simulink model "All_Controller_Compare_Angle_Disturbance"  (R2022a)
settings: Solver=VariableStepAuto  StartTime=0.0  StopTime=130  RelTol=1e-3
undefined symbols (not defined in the file): A, att_opt, B, C, ki_u4_, Klqr, L, pitch_opt, roll_opt, x_opt, y_opt, yaw_opt
libraries: slpidlib x6, simulink x2
settings Model: Creator=creec  LastModifiedBy=creec

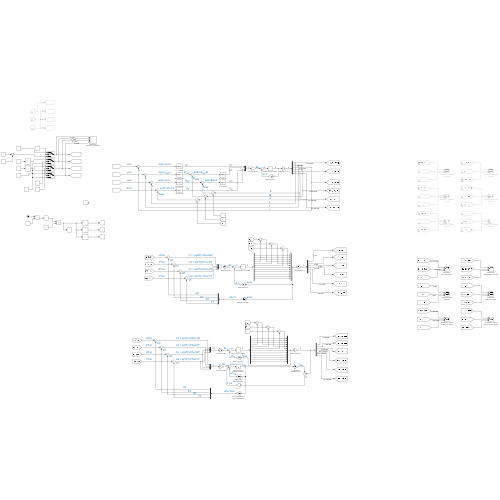
[thumbnail: Simulink's stored preview of the top-level diagram]
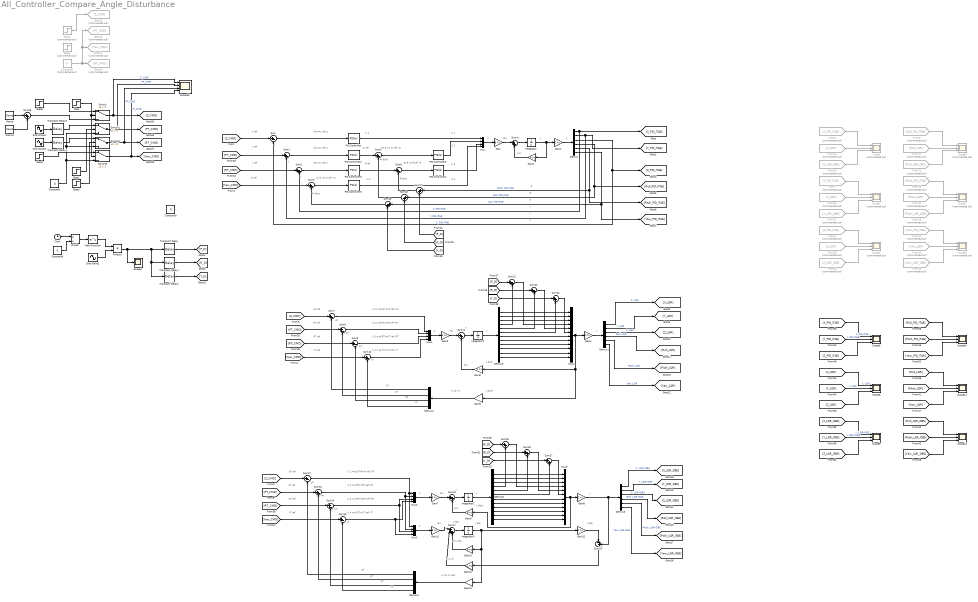
== system All_Controller_Compare_Angle_Disturbance ==
  note: z
  note: x ref
  note: U 1
  note: U 4
  note: x
  note: Ψ distr
  note: x'
  note: θ
  note: Ψ ref
  note: e(y)=y ref -y
  note: e(x)=x ref -x
  note: U 1
  note: e( θ )= θ ref - θ
  note: Φ ref
  note: x
  note: x
  note: Ψ
  note: A*x
  note: e(z)=z ref -z
  note: y
  note: U 2
  note: U
  note: z
  note: θ distr
  note: Bu
  note: U 4
  note: Φ distr
  note: Φ
  note: y ref
  note: y
  note: y
  note: z ref
  note: e( Ψ )= Ψ ref - Ψ
  note: U 3
  note: θ ref
  note: e( Φ )= Φ ref - Φ
  note: PT
  note: y
  note: U 3 = e(RT)=RT ref -RT
  note: U 4 = e(YT)=YT ref -YT
  note: U 2 = e(PT)=PT ref -PT
  note: x distr
  note: RT
  note: PT
  note: - K lqr *x
  note: UF
  note: Bu
  note: UF ref
  note: U 1 = e(UF)=UF ref -UF
  note: RT ref
  note: x
  note: UF
  note: A*x
  note: YT ref
  note: PT ref
  note: U
  note: x'
  note: YT
  note: RT
  note: YT
  note: x obs
  note: L*y e
  note: RT ref
  note: YT ref
  note: x
  note: U
  note: YT
  note: U 1 = e(UF)=UF ref -UF
  note: x'
  note: A*x
  note: YT
  note: A*x obs
  note: PT ref
  note: UF
  note: U
  note: UF
  note: UF ref
  note: Bu
  note: RT
  note: U 2 = e(PT)=PT ref -PT
  note: RT
  note: U 4 = e(YT)=YT ref -YT
  note: x obs '
  note: PT
  note: U 3 = e(RT)=RT ref -RT
  note: PT
  note: y e
  note: - K lqr *x obs
  note: y
  note: y obs
  note: Bu
  note: x distr
  note: x distr
  Clock : Clock
  Constant1 : Constant  Value=0
  Constant6 : Constant  Commented=on  Value=0
  Constant8 : Constant  Value=-1  SampleTime=-1
  Constant9 : Constant  Value=0
  Demux : Demux  Outputs=6
  Demux1 : Demux  Outputs=6
  Demux2 : Demux
  Demux3 : Demux  Outputs=6
  Demux4 : Demux
  Demux5 : Demux  Outputs=12
  Demux6 : Demux  Outputs=12
  Divide : Product  Inputs=*/
  From10 : From  Commented=on  GotoTag=Pitch_PID_ITAE
  From11 : From  Commented=on  GotoTag=Yaw_PID_ITAE
  From12 : From  Commented=on  GotoTag=Pitch_LQR
  From13 : From  Commented=on  GotoTag=Yaw_LQR
  From14 : From  Commented=on  GotoTag=X_LQR
  From15 : From  Commented=on  GotoTag=Y_LQR
  From16 : From  Commented=on  GotoTag=Z_LQR
  From17 : From  Commented=on  GotoTag=Roll_LQR
  From18 : From  Commented=on  GotoTag=Pitch_LQR_OBS
  From19 : From  Commented=on  GotoTag=Yaw_LQR_OBS
  From20 : From  Commented=on  GotoTag=X_LQR_OBS
  From21 : From  Commented=on  GotoTag=Y_LQR_OBS
  From22 : From  Commented=on  GotoTag=Z_LQR_OBS
  From23 : From  Commented=on  GotoTag=Roll_LQR_OBS
  From6 : From  Commented=on  GotoTag=X_PID_ITAE
  From7 : From  Commented=on  GotoTag=Y_PID_ITAE
  From8 : From  Commented=on  GotoTag=Z_PID_ITAE
  From9 : From  Commented=on  GotoTag=Roll_PID_ITAE
  Gain{,3,7,11} (4 alike) : Gain  Gain=B  Multiplication=Matrix(K*u)
      settings: AttributesFormatString=State-Space B*u
  Gain{1,4,8,12} (4 alike) : Gain  Gain=C  Multiplication=Matrix(K*u)
      Gain1 settings: AttributesFormatString=State-Space C*x
      Gain12 settings: AttributesFormatString=|
      | Augmented
      | State-Space C*x
      Gain4 settings: AttributesFormatString=State-Space C*x
      Gain8 settings: AttributesFormatString=State-Space C*x
  Gain10 : Gain  Gain=Klqr  Multiplication=Matrix(K*u)
      settings: AttributesFormatString=|
      | LQR Feedback Gain,
      | Augmented States
  Gain{2,5,9,13} (4 alike) : Gain  Gain=A  Multiplication=Matrix(K*u)
      Gain13 settings: AttributesFormatString=|
      | Augmented
      | State-Space A*x
      Gain2 settings: AttributesFormatString=State-Space A*x
      Gain5 settings: AttributesFormatString=State-Space A*x
      Gain9 settings: AttributesFormatString=State-Space A*x
  Gain14 : Gain  Gain=L  Multiplication=Matrix(K*u)
      settings: AttributesFormatString=L*y_e
  Gain6 : Gain  Gain=Klqr  Multiplication=Matrix(K*u)
      settings: AttributesFormatString=LQR Feeback Gain
  Goto21 : Goto  Commented=on  GotoTag=Yaw_CMD
  Goto23 : Goto  Commented=on  GotoTag=PT_CMD
  Goto24 : Goto  Commented=on  GotoTag=RT_CMD
  Goto25 : Goto  Commented=on  GotoTag=Z_CMD
  Integrator{,1..3} (4 alike) : Integrator
      Integrator settings: AttributesFormatString=Extract Current States
      Integrator1 settings: AttributesFormatString=Extract Current States
      Integrator2 settings: AttributesFormatString=Extract Current States
      Integrator3 settings: AttributesFormatString=|
      | Extract Current
      | Augmented States
  Math Function : Math
  Mux{,1..3} (4 alike) : Mux
  Mux4 : Mux  Inputs=12
  Mux5 : Mux  Inputs=12
  PID Controller : slpidlib/PID Controller  Controller=PID  Form=Parallel  TimeDomain=Continuous-time  UseExternalTs=off  SampleTime=-1  IntegratorMethod=Forward Euler  FilterMethod=Forward Euler  ControllerParametersSource=internal  P=att_opt(1)  I=att_opt(2)  UseKiTs=off  D=att_opt(3)  N=100  UseFilter=on  TunerSelectOption=Transfer Function Based (PID Tuner App)  InitialConditionSource=internal  InitialConditionForIntegrator=0  InitialConditionForFilter=0  DifferentiatorICPrevScaledInput=0  ExternalReset=none  TrackingMode=off  Kt=1  LimitOutput=off  SatLimitsSource=internal  UpperSaturationLimit=inf  LowerSaturationLimit=-inf  LinearizeAsGain=on  AntiWindupMode=none  Kb=1  POutMin=[]  POutMax=[]  IOutMin=[]  IOutMax=[]  DOutMin=[]  DOutMax=[]  NOutMin=[]  NOutMax=[]  SumOutMin=[]  SumOutMax=[]  SaturationOutMin=[]  SaturationOutMax=[]  PParamMin=[]  PParamMax=[]  IParamMin=[]  IParamMax=[]  DParamMin=[]  DParamMax=[]  NParamMin=[]  NParamMax=[]  KbParamMin=[]  KbParamMax=[]  KtParamMin=[]  KtParamMax=[]  KbOutMin=[]  KbOutMax=[]  KtOutMin=[]  KtOutMax=[]  IntegratorOutMin=[]  IntegratorOutMax=[]  FilterOutMin=[]  FilterOutMax=[]  SumI1OutMin=[]  SumI1OutMax=[]  SumI2OutMin=[]  SumI2OutMax=[]  SumI3OutMin=[]  SumI3OutMax=[]  SumI4OutMin=[]  SumI4OutMax=[]  SumDOutMin=[]  SumDOutMax=[]  DifferentiatorOutMin=[]  DifferentiatorOutMax=[]  FilterDiffOutCoefMin=[]  FilterDiffOutCoefMax=[]  ReciprocalOutMin=[]  ReciprocalOutMax=[]  SumDenOutMin=[]  SumDenOutMax=[]  SumNumOutMin=[]  SumNumOutMax=[]  DivideOutMin=[]  DivideOutMax=[]  UdiffTsProdOutMin=[]  UdiffTsProdOutMax=[]  NTsProdOutMin=[]  NTsProdOutMax=[]  UintegralTsProdOutMin=[]  UintegralTsProdOutMax=[]  UngainTsProdOutMin=[]  UngainTsProdOutMax=[]  IntegratorContinuousStateAttributes=''  IntegratorStateMustResolveToSignalObject=off  IntegratorRTWStateStorageClass=Auto  FilterContinuousStateAttributes=''  FilterStateMustResolveToSignalObject=off  FilterRTWStateStorageClass=Auto  ParallelPVariant=InternalParameters  IdealPVariant=Disabled  IVariant=InternalParameters  DVariant=InternalParameters  IntegratorVariant=Continuous  SatVariant=Disabled  AWVariant=Passthrough  PCopyVariant=Disabled  TRVariant=Disabled  FdbkBlocksVariant=Forward  IdealPFdbkVariant=Disabled  SatFdbkVariant=Disabled  DerivativeFilterVariant=ContFilter  NVariant=InternalParameters  NCopyVariant=Disabled  FilterICVariant=InternalICsFilter  IntegratorICVariant=InternalICs  ExternalResetVariant=Disabled  TRSumVariant=Passthrough  SumFdbkVariant=Disabled  SumVariant=Sum_PID  TsampFilterVariant=InternalTs  TsampNgainVariant=Passthrough  TsampIntegralVariant=Passthrough  ExternalSaturationOutDataTypeStr=Inherit: Same as second input  aMode=0
      settings: AttributesFormatString=U1 Controller
  PID Controller1 : slpidlib/PID Controller  Controller=PD  Form=Parallel  TimeDomain=Continuous-time  UseExternalTs=off  SampleTime=-1  IntegratorMethod=Forward Euler  FilterMethod=Forward Euler  ControllerParametersSource=internal  P=y_opt(1)  I=0  UseKiTs=off  D=y_opt(2)  N=100  UseFilter=on  TunerSelectOption=Transfer Function Based (PID Tuner App)  InitialConditionSource=internal  InitialConditionForIntegrator=0  InitialConditionForFilter=0  DifferentiatorICPrevScaledInput=0  ExternalReset=none  TrackingMode=off  Kt=1  LimitOutput=off  SatLimitsSource=internal  UpperSaturationLimit=inf  LowerSaturationLimit=-inf  LinearizeAsGain=on  AntiWindupMode=none  Kb=1  POutMin=[]  POutMax=[]  IOutMin=[]  IOutMax=[]  DOutMin=[]  DOutMax=[]  NOutMin=[]  NOutMax=[]  SumOutMin=[]  SumOutMax=[]  SaturationOutMin=[]  SaturationOutMax=[]  PParamMin=[]  PParamMax=[]  IParamMin=[]  IParamMax=[]  DParamMin=[]  DParamMax=[]  NParamMin=[]  NParamMax=[]  KbParamMin=[]  KbParamMax=[]  KtParamMin=[]  KtParamMax=[]  KbOutMin=[]  KbOutMax=[]  KtOutMin=[]  KtOutMax=[]  IntegratorOutMin=[]  IntegratorOutMax=[]  FilterOutMin=[]  FilterOutMax=[]  SumI1OutMin=[]  SumI1OutMax=[]  SumI2OutMin=[]  SumI2OutMax=[]  SumI3OutMin=[]  SumI3OutMax=[]  SumI4OutMin=[]  SumI4OutMax=[]  SumDOutMin=[]  SumDOutMax=[]  DifferentiatorOutMin=[]  DifferentiatorOutMax=[]  FilterDiffOutCoefMin=[]  FilterDiffOutCoefMax=[]  ReciprocalOutMin=[]  ReciprocalOutMax=[]  SumDenOutMin=[]  SumDenOutMax=[]  SumNumOutMin=[]  SumNumOutMax=[]  DivideOutMin=[]  DivideOutMax=[]  UdiffTsProdOutMin=[]  UdiffTsProdOutMax=[]  NTsProdOutMin=[]  NTsProdOutMax=[]  UintegralTsProdOutMin=[]  UintegralTsProdOutMax=[]  UngainTsProdOutMin=[]  UngainTsProdOutMax=[]  IntegratorContinuousStateAttributes=''  IntegratorStateMustResolveToSignalObject=off  IntegratorRTWStateStorageClass=Auto  FilterContinuousStateAttributes=''  FilterStateMustResolveToSignalObject=off  FilterRTWStateStorageClass=Auto  ParallelPVariant=InternalParameters  IdealPVariant=Disabled  IVariant=Disabled  DVariant=InternalParameters  IntegratorVariant=Disabled  SatVariant=Disabled  AWVariant=Disabled  PCopyVariant=Disabled  TRVariant=Disabled  FdbkBlocksVariant=Forward  IdealPFdbkVariant=Disabled  SatFdbkVariant=Disabled  DerivativeFilterVariant=ContFilter  NVariant=InternalParameters  NCopyVariant=Disabled  FilterICVariant=InternalICsFilter  IntegratorICVariant=Disabled  ExternalResetVariant=Disabled  TRSumVariant=Passthrough  SumFdbkVariant=Disabled  SumVariant=Sum_PD  TsampFilterVariant=InternalTs  TsampNgainVariant=Passthrough  TsampIntegralVariant=Disabled_SignalSpec  ExternalSaturationOutDataTypeStr=Inherit: Same as second input  aMode=0
      settings: AttributesFormatString=Φref Generation
  PID Controller2 : slpidlib/PID Controller  Controller=PID  Form=Parallel  TimeDomain=Continuous-time  UseExternalTs=off  SampleTime=-1  IntegratorMethod=Forward Euler  FilterMethod=Forward Euler  ControllerParametersSource=internal  P=pitch_opt(1)  I=pitch_opt(2)  UseKiTs=off  D=pitch_opt(3)  N=100  UseFilter=on  TunerSelectOption=Transfer Function Based (PID Tuner App)  InitialConditionSource=internal  InitialConditionForIntegrator=0  InitialConditionForFilter=0  DifferentiatorICPrevScaledInput=0  ExternalReset=none  TrackingMode=off  Kt=1  LimitOutput=off  SatLimitsSource=internal  UpperSaturationLimit=inf  LowerSaturationLimit=-inf  LinearizeAsGain=on  AntiWindupMode=none  Kb=1  POutMin=[]  POutMax=[]  IOutMin=[]  IOutMax=[]  DOutMin=[]  DOutMax=[]  NOutMin=[]  NOutMax=[]  SumOutMin=[]  SumOutMax=[]  SaturationOutMin=[]  SaturationOutMax=[]  PParamMin=[]  PParamMax=[]  IParamMin=[]  IParamMax=[]  DParamMin=[]  DParamMax=[]  NParamMin=[]  NParamMax=[]  KbParamMin=[]  KbParamMax=[]  KtParamMin=[]  KtParamMax=[]  KbOutMin=[]  KbOutMax=[]  KtOutMin=[]  KtOutMax=[]  IntegratorOutMin=[]  IntegratorOutMax=[]  FilterOutMin=[]  FilterOutMax=[]  SumI1OutMin=[]  SumI1OutMax=[]  SumI2OutMin=[]  SumI2OutMax=[]  SumI3OutMin=[]  SumI3OutMax=[]  SumI4OutMin=[]  SumI4OutMax=[]  SumDOutMin=[]  SumDOutMax=[]  DifferentiatorOutMin=[]  DifferentiatorOutMax=[]  FilterDiffOutCoefMin=[]  FilterDiffOutCoefMax=[]  ReciprocalOutMin=[]  ReciprocalOutMax=[]  SumDenOutMin=[]  SumDenOutMax=[]  SumNumOutMin=[]  SumNumOutMax=[]  DivideOutMin=[]  DivideOutMax=[]  UdiffTsProdOutMin=[]  UdiffTsProdOutMax=[]  NTsProdOutMin=[]  NTsProdOutMax=[]  UintegralTsProdOutMin=[]  UintegralTsProdOutMax=[]  UngainTsProdOutMin=[]  UngainTsProdOutMax=[]  IntegratorContinuousStateAttributes=''  IntegratorStateMustResolveToSignalObject=off  IntegratorRTWStateStorageClass=Auto  FilterContinuousStateAttributes=''  FilterStateMustResolveToSignalObject=off  FilterRTWStateStorageClass=Auto  ParallelPVariant=InternalParameters  IdealPVariant=Disabled  IVariant=InternalParameters  DVariant=InternalParameters  IntegratorVariant=Continuous  SatVariant=Disabled  AWVariant=Passthrough  PCopyVariant=Disabled  TRVariant=Disabled  FdbkBlocksVariant=Forward  IdealPFdbkVariant=Disabled  SatFdbkVariant=Disabled  DerivativeFilterVariant=ContFilter  NVariant=InternalParameters  NCopyVariant=Disabled  FilterICVariant=InternalICsFilter  IntegratorICVariant=InternalICs  ExternalResetVariant=Disabled  TRSumVariant=Passthrough  SumFdbkVariant=Disabled  SumVariant=Sum_PID  TsampFilterVariant=InternalTs  TsampNgainVariant=Passthrough  TsampIntegralVariant=Passthrough  ExternalSaturationOutDataTypeStr=Inherit: Same as second input  aMode=0
      settings: AttributesFormatString=U2 Controller
  PID Controller3 : slpidlib/PID Controller  Controller=PD  Form=Parallel  TimeDomain=Continuous-time  UseExternalTs=off  SampleTime=-1  IntegratorMethod=Forward Euler  FilterMethod=Forward Euler  ControllerParametersSource=internal  P=x_opt(1)  I=-0.0096  UseKiTs=off  D=x_opt(2)  N=100  UseFilter=on  TunerSelectOption=Transfer Function Based (PID Tuner App)  InitialConditionSource=internal  InitialConditionForIntegrator=0  InitialConditionForFilter=0  DifferentiatorICPrevScaledInput=0  ExternalReset=none  TrackingMode=off  Kt=1  LimitOutput=off  SatLimitsSource=internal  UpperSaturationLimit=inf  LowerSaturationLimit=-inf  LinearizeAsGain=on  AntiWindupMode=none  Kb=1  POutMin=[]  POutMax=[]  IOutMin=[]  IOutMax=[]  DOutMin=[]  DOutMax=[]  NOutMin=[]  NOutMax=[]  SumOutMin=[]  SumOutMax=[]  SaturationOutMin=[]  SaturationOutMax=[]  PParamMin=[]  PParamMax=[]  IParamMin=[]  IParamMax=[]  DParamMin=[]  DParamMax=[]  NParamMin=[]  NParamMax=[]  KbParamMin=[]  KbParamMax=[]  KtParamMin=[]  KtParamMax=[]  KbOutMin=[]  KbOutMax=[]  KtOutMin=[]  KtOutMax=[]  IntegratorOutMin=[]  IntegratorOutMax=[]  FilterOutMin=[]  FilterOutMax=[]  SumI1OutMin=[]  SumI1OutMax=[]  SumI2OutMin=[]  SumI2OutMax=[]  SumI3OutMin=[]  SumI3OutMax=[]  SumI4OutMin=[]  SumI4OutMax=[]  SumDOutMin=[]  SumDOutMax=[]  DifferentiatorOutMin=[]  DifferentiatorOutMax=[]  FilterDiffOutCoefMin=[]  FilterDiffOutCoefMax=[]  ReciprocalOutMin=[]  ReciprocalOutMax=[]  SumDenOutMin=[]  SumDenOutMax=[]  SumNumOutMin=[]  SumNumOutMax=[]  DivideOutMin=[]  DivideOutMax=[]  UdiffTsProdOutMin=[]  UdiffTsProdOutMax=[]  NTsProdOutMin=[]  NTsProdOutMax=[]  UintegralTsProdOutMin=[]  UintegralTsProdOutMax=[]  UngainTsProdOutMin=[]  UngainTsProdOutMax=[]  IntegratorContinuousStateAttributes=''  IntegratorStateMustResolveToSignalObject=off  IntegratorRTWStateStorageClass=Auto  FilterContinuousStateAttributes=''  FilterStateMustResolveToSignalObject=off  FilterRTWStateStorageClass=Auto  ParallelPVariant=InternalParameters  IdealPVariant=Disabled  IVariant=Disabled  DVariant=InternalParameters  IntegratorVariant=Disabled  SatVariant=Disabled  AWVariant=Disabled  PCopyVariant=Disabled  TRVariant=Disabled  FdbkBlocksVariant=Forward  IdealPFdbkVariant=Disabled  SatFdbkVariant=Disabled  DerivativeFilterVariant=ContFilter  NVariant=InternalParameters  NCopyVariant=Disabled  FilterICVariant=InternalICsFilter  IntegratorICVariant=Disabled  ExternalResetVariant=Disabled  TRSumVariant=Passthrough  SumFdbkVariant=Disabled  SumVariant=Sum_PD  TsampFilterVariant=InternalTs  TsampNgainVariant=Passthrough  TsampIntegralVariant=Disabled_SignalSpec  ExternalSaturationOutDataTypeStr=Inherit: Same as second input  aMode=0
      settings: AttributesFormatString=θref Generation
  PID Controller4 : slpidlib/PID Controller  Controller=PID  Form=Parallel  TimeDomain=Continuous-time  UseExternalTs=off  SampleTime=-1  IntegratorMethod=Forward Euler  FilterMethod=Forward Euler  ControllerParametersSource=internal  P=roll_opt(1)  I=roll_opt(2)  UseKiTs=off  D=roll_opt(3)  N=100  UseFilter=on  TunerSelectOption=Transfer Function Based (PID Tuner App)  InitialConditionSource=internal  InitialConditionForIntegrator=0  InitialConditionForFilter=0  DifferentiatorICPrevScaledInput=0  ExternalReset=none  TrackingMode=off  Kt=1  LimitOutput=off  SatLimitsSource=internal  UpperSaturationLimit=inf  LowerSaturationLimit=-inf  LinearizeAsGain=on  AntiWindupMode=none  Kb=1  POutMin=[]  POutMax=[]  IOutMin=[]  IOutMax=[]  DOutMin=[]  DOutMax=[]  NOutMin=[]  NOutMax=[]  SumOutMin=[]  SumOutMax=[]  SaturationOutMin=[]  SaturationOutMax=[]  PParamMin=[]  PParamMax=[]  IParamMin=[]  IParamMax=[]  DParamMin=[]  DParamMax=[]  NParamMin=[]  NParamMax=[]  KbParamMin=[]  KbParamMax=[]  KtParamMin=[]  KtParamMax=[]  KbOutMin=[]  KbOutMax=[]  KtOutMin=[]  KtOutMax=[]  IntegratorOutMin=[]  IntegratorOutMax=[]  FilterOutMin=[]  FilterOutMax=[]  SumI1OutMin=[]  SumI1OutMax=[]  SumI2OutMin=[]  SumI2OutMax=[]  SumI3OutMin=[]  SumI3OutMax=[]  SumI4OutMin=[]  SumI4OutMax=[]  SumDOutMin=[]  SumDOutMax=[]  DifferentiatorOutMin=[]  DifferentiatorOutMax=[]  FilterDiffOutCoefMin=[]  FilterDiffOutCoefMax=[]  ReciprocalOutMin=[]  ReciprocalOutMax=[]  SumDenOutMin=[]  SumDenOutMax=[]  SumNumOutMin=[]  SumNumOutMax=[]  DivideOutMin=[]  DivideOutMax=[]  UdiffTsProdOutMin=[]  UdiffTsProdOutMax=[]  NTsProdOutMin=[]  NTsProdOutMax=[]  UintegralTsProdOutMin=[]  UintegralTsProdOutMax=[]  UngainTsProdOutMin=[]  UngainTsProdOutMax=[]  IntegratorContinuousStateAttributes=''  IntegratorStateMustResolveToSignalObject=off  IntegratorRTWStateStorageClass=Auto  FilterContinuousStateAttributes=''  FilterStateMustResolveToSignalObject=off  FilterRTWStateStorageClass=Auto  ParallelPVariant=InternalParameters  IdealPVariant=Disabled  IVariant=InternalParameters  DVariant=InternalParameters  IntegratorVariant=Continuous  SatVariant=Disabled  AWVariant=Passthrough  PCopyVariant=Disabled  TRVariant=Disabled  FdbkBlocksVariant=Forward  IdealPFdbkVariant=Disabled  SatFdbkVariant=Disabled  DerivativeFilterVariant=ContFilter  NVariant=InternalParameters  NCopyVariant=Disabled  FilterICVariant=InternalICsFilter  IntegratorICVariant=InternalICs  ExternalResetVariant=Disabled  TRSumVariant=Passthrough  SumFdbkVariant=Disabled  SumVariant=Sum_PID  TsampFilterVariant=InternalTs  TsampNgainVariant=Passthrough  TsampIntegralVariant=Passthrough  ExternalSaturationOutDataTypeStr=Inherit: Same as second input  aMode=0
      settings: AttributesFormatString=U3 Controller
  PID Controller5 : slpidlib/PID Controller  Controller=PD  Form=Parallel  TimeDomain=Continuous-time  UseExternalTs=off  SampleTime=-1  IntegratorMethod=Forward Euler  FilterMethod=Forward Euler  ControllerParametersSource=internal  P=yaw_opt(1)  I=ki_u4_  UseKiTs=off  D=yaw_opt(2)  N=100  UseFilter=on  TunerSelectOption=Transfer Function Based (PID Tuner App)  InitialConditionSource=internal  InitialConditionForIntegrator=0  InitialConditionForFilter=0  DifferentiatorICPrevScaledInput=0  ExternalReset=none  TrackingMode=off  Kt=1  LimitOutput=off  SatLimitsSource=internal  UpperSaturationLimit=inf  LowerSaturationLimit=-inf  LinearizeAsGain=on  AntiWindupMode=none  Kb=1  POutMin=[]  POutMax=[]  IOutMin=[]  IOutMax=[]  DOutMin=[]  DOutMax=[]  NOutMin=[]  NOutMax=[]  SumOutMin=[]  SumOutMax=[]  SaturationOutMin=[]  SaturationOutMax=[]  PParamMin=[]  PParamMax=[]  IParamMin=[]  IParamMax=[]  DParamMin=[]  DParamMax=[]  NParamMin=[]  NParamMax=[]  KbParamMin=[]  KbParamMax=[]  KtParamMin=[]  KtParamMax=[]  KbOutMin=[]  KbOutMax=[]  KtOutMin=[]  KtOutMax=[]  IntegratorOutMin=[]  IntegratorOutMax=[]  FilterOutMin=[]  FilterOutMax=[]  SumI1OutMin=[]  SumI1OutMax=[]  SumI2OutMin=[]  SumI2OutMax=[]  SumI3OutMin=[]  SumI3OutMax=[]  SumI4OutMin=[]  SumI4OutMax=[]  SumDOutMin=[]  SumDOutMax=[]  DifferentiatorOutMin=[]  DifferentiatorOutMax=[]  FilterDiffOutCoefMin=[]  FilterDiffOutCoefMax=[]  ReciprocalOutMin=[]  ReciprocalOutMax=[]  SumDenOutMin=[]  SumDenOutMax=[]  SumNumOutMin=[]  SumNumOutMax=[]  DivideOutMin=[]  DivideOutMax=[]  UdiffTsProdOutMin=[]  UdiffTsProdOutMax=[]  NTsProdOutMin=[]  NTsProdOutMax=[]  UintegralTsProdOutMin=[]  UintegralTsProdOutMax=[]  UngainTsProdOutMin=[]  UngainTsProdOutMax=[]  IntegratorContinuousStateAttributes=''  IntegratorStateMustResolveToSignalObject=off  IntegratorRTWStateStorageClass=Auto  FilterContinuousStateAttributes=''  FilterStateMustResolveToSignalObject=off  FilterRTWStateStorageClass=Auto  ParallelPVariant=InternalParameters  IdealPVariant=Disabled  IVariant=Disabled  DVariant=InternalParameters  IntegratorVariant=Disabled  SatVariant=Disabled  AWVariant=Disabled  PCopyVariant=Disabled  TRVariant=Disabled  FdbkBlocksVariant=Forward  IdealPFdbkVariant=Disabled  SatFdbkVariant=Disabled  DerivativeFilterVariant=ContFilter  NVariant=InternalParameters  NCopyVariant=Disabled  FilterICVariant=InternalICsFilter  IntegratorICVariant=Disabled  ExternalResetVariant=Disabled  TRSumVariant=Passthrough  SumFdbkVariant=Disabled  SumVariant=Sum_PD  TsampFilterVariant=InternalTs  TsampNgainVariant=Passthrough  TsampIntegralVariant=Disabled_SignalSpec  ExternalSaturationOutDataTypeStr=Inherit: Same as second input  aMode=0
      settings: AttributesFormatString=U4 Controller
  Product : Product
  Ramp : simulink/Sources/Ramp  slope=-0.4  start=58.46+40  InitialOutput=8
  Ramp1 : simulink/Sources/Ramp  slope=0.4  start=58.46+60  InitialOutput=0
  Scope{,1..3,7..8} (6 alike) : Scope  Commented=on  NumInputPorts=3
      Scope settings: AttributesFormatString=|
      | Quadcopter X-Position
      | Outputs
      Scope1 settings: AttributesFormatString=|
      | Quadcopter Y-Position
      | Outputs
      Scope2 settings: AttributesFormatString=|
      | Quadcopter Z-Position
      | Outputs
      Scope3 settings: AttributesFormatString=|
      | Quadcopter Roll Angle
      | Outputs
      Scope7 settings: AttributesFormatString=|
      | Quadcopter Pitch Angle
      | Outputs
      Scope8 settings: AttributesFormatString=|
      | Quadcopter Yaw Angle
      | Outputs
  Scope{5..6,9..12} (6 alike) : Scope  NumInputPorts=3
      Scope10 settings: AttributesFormatString=|
      | Quadcopter
      | PID-ITAE Euler Angles
      Scope11 settings: AttributesFormatString=|
      | Quadcopter
      | LQR Euler Angles
      Scope12 settings: AttributesFormatString=|
      | Quadcopter LQR-PI
      | (Observer) Euler Angles
      Scope5 settings: AttributesFormatString=|
      | Quadcopter
      | PID-ITAE Positions
      Scope6 settings: AttributesFormatString=|
      | Quadcopter LQR
      | Positions
      Scope9 settings: AttributesFormatString=|
      | Quadcopter LQR-PI
      | (Observer) Positions
  Scope13 : Scope  NumInputPorts=4
      settings: AttributesFormatString=|
      | Quadcopter
      | Reference Commands
  Scope4 : Scope
  Sine Wave1 : Sin  Amplitude=5  Frequency=0.3142  SampleTime=0
  Sine Wave2 : Sin  Amplitude=0.4  Bias=0.2  Frequency=62.83185  SampleTime=0
  Sine Wave3 : Sin  Amplitude=5  Frequency=0.3142  Phase=pi/2  SampleTime=0
  Step : Step  Time=58.46+40  Before=1  After=0  SampleTime=0
  Step1 : Step  Time=94.2  Before=1  After=0  SampleTime=0
  Step2 : Step  After=0.25  SampleTime=0
  Step3 : Step  Time=99.285  Before=1  After=0  SampleTime=0
  Step4 : Step  Commented=on  Time=0  After=5  SampleTime=0
  Step5 : Step  Commented=on  After=8  SampleTime=0
  Step6 : Step  Time=0  After=8  SampleTime=0
  Sum{,1,3,5..10,12..15} (13 alike) : Sum  Inputs=|+-
  Sum{2,4,11,16,19..28} (14 alike) : Sum  Inputs=|++
  Sum17 : Sum  Inputs=|+++
  Sum18 : Sum  Inputs=|-+
  Switch{,1..3} (4 alike) : Switch  Criteria=u2 > Threshold  SaturateOnIntegerOverflow=off  InputSameDT=off
  Transport Delay : TransportDelay  DelayTime=5+20
  Transport Delay1 : TransportDelay  DelayTime=10+20
  Transport Delay2 : TransportDelay  DelayTime=7
  Transport Delay3 : TransportDelay  DelayTime=12.5
  Transport Delay4 : TransportDelay  DelayTime=12.5
  wires:
  Demux/1 -> [X_PID_ITAE], Sum2/2  "X, PID-ITAE"
  Demux/2 -> [Y_PID_ITAE], Sum1/2  "Y, PID-ITAE"
  [PT_CMD] -> Sum1/1
  Demux/5 -> Sum21/1, [Pitch_PID_ITAE]  "Pitch, PID-ITAE"
  [RT_CMD] -> Sum2/1
  PID Controller5/1 -> Mux/4
  [Yaw_CMD] -> Sum3/1
  Sum6/1 -> PID Controller4/1
  PID Controller3/1 -> Sum6/1
  [Z_CMD] -> Sum/1
  PID Controller/1 -> Mux/1
  Mux/1 -> Gain/1
  Demux/4 -> Sum20/1, [Roll_PID_ITAE]  "Roll, PID-ITAE"
  Demux/3 -> [Z_PID_ITAE], Sum/2  "Z, PID-ITAE"
  Demux/6 -> Sum19/1, [Yaw_PID_ITAE]  "Yaw, PID-ITAE"
  Sum5/1 -> PID Controller2/1
  Integrator/1 -> Gain2/1, Gain1/1
  Sum2/1 -> PID Controller3/1
  Sum1/1 -> PID Controller1/1
  PID Controller1/1 -> Sum5/1
  Sum4/1 -> Integrator/1
  Sum/1 -> PID Controller/1
  PID Controller4/1 -> Mux/3
  Gain2/1 -> Sum4/2
  PID Controller2/1 -> Mux/2
  Sum3/1 -> PID Controller5/1
  Gain/1 -> Sum4/1
  Gain1/1 -> Demux/1
  Gain4/1 -> Demux1/1
  Sum8/1 -> Mux1/2
  Demux2/3 -> Sum9/2
  Sum9/1 -> Mux1/3
  Demux2/2 -> Sum8/2
  Demux1/5 -> [Pitch_LQR]  "Pitch, LQR"
  [PT_CMD] -> Sum8/1
  [RT_CMD] -> Sum9/1
  Gain6/1 -> Demux2/1
  Demux1/6 -> [Yaw_LQR]  "Yaw, LQR"
  [Yaw_CMD] -> Sum10/1
  Gain3/1 -> Sum11/1
  Demux2/1 -> Sum7/2
  Sum10/1 -> Mux1/4
  Demux1/1 -> [X_LQR]  "X, LQR"
  Demux1/3 -> [Z_LQR]  "Z, LQR"
  Gain5/1 -> Sum11/2
  Demux1/4 -> [Roll_LQR]  "Roll, LQR"
  Integrator1/1 -> Demux5/1
  Mux1/1 -> Gain3/1
  Demux1/2 -> [Y_LQR]  "Y, LQR"
  Demux2/4 -> Sum10/2
  [Z_CMD] -> Sum7/1
  Sum7/1 -> Mux1/1
  Sum11/1 -> Integrator1/1
  Gain14/1 -> Sum17/2
  Integrator3/1 -> Gain10/1, Gain13/1, Gain12/1
  Sum17/1 -> Integrator3/1
  Demux4/4 -> Sum15/2
  [Z_CMD] -> Sum12/1
  Sum12/1 -> Mux3/1, Mux2/1
  Gain11/1 -> Sum17/1
  Integrator2/1 -> Demux6/1
  Mux2/1 -> Gain7/1
  Sum16/1 -> Integrator2/1
  Demux4/2 -> Sum13/2
  [Yaw_CMD] -> Sum15/1
  Gain9/1 -> Sum16/2
  Gain7/1 -> Sum16/1
  Demux3/5 -> [Pitch_LQR_OBS]  "Pitch, LQR-OBS"
  Sum15/1 -> Mux2/4, Mux3/4
  [PT_CMD] -> Sum13/1
  Demux4/1 -> Sum12/2
  Sum14/1 -> Mux2/3, Mux3/3
  Demux4/3 -> Sum14/2
  Gain8/1 -> Sum18/2, Demux3/1
  Sum13/1 -> Mux2/2, Mux3/2
  [RT_CMD] -> Sum14/1
  Gain13/1 -> Sum17/3
  Mux3/1 -> Gain11/1
  Sum18/1 -> Gain14/1
  Gain10/1 -> Demux4/1
  Demux3/4 -> [Roll_LQR_OBS]  "Roll, LQR-OBS"
  Demux3/3 -> [Z_LQR_OBS]  "Z, LQR-OBS"
  Demux3/2 -> [Y_LQR_OBS]  "Y, LQR-OBS"
  Demux3/6 -> [Yaw_LQR_OBS]  "Yaw, LQR-OBS"
  Gain12/1 -> Sum18/1
  Demux3/1 -> [X_LQR_OBS]  "X, LQR-OBS"
  From6/1 -> Scope/1
  From14/1 -> Scope/2
  From20/1 -> Scope/3
  From15/1 -> Scope1/2
  From7/1 -> Scope1/1
  From21/1 -> Scope1/3
  From8/1 -> Scope2/1
  From16/1 -> Scope2/2
  From22/1 -> Scope2/3
  From11/1 -> Scope8/1
  From23/1 -> Scope3/3
  From10/1 -> Scope7/1
  From17/1 -> Scope3/2
  From13/1 -> Scope8/2
  From12/1 -> Scope7/2
  From19/1 -> Scope8/3
  From18/1 -> Scope7/3
  From9/1 -> Scope3/1
  Constant8/1 -> Divide/2
  Clock/1 -> Divide/1
  Sine Wave2/1 -> Product/2
  Math Function/1 -> Product/1
  Divide/1 -> Math Function/1
  Product/1 -> Transport Delay2/1, Transport Delay1/1, Transport Delay/1, Scope4/1
  Sum19/1 -> Sum3/2
  Sum20/1 -> Sum5/2
  Sum21/1 -> Sum6/2
  [P_D] -> Sum21/2
  [R_D] -> Sum20/2
  [Y_D] -> Sum19/2
  [R_D] -> Sum23/1
  Sum23/1 -> Mux4/5
  Demux5/11 -> Mux4/11
  Demux5/9 -> Mux4/9
  Demux5/10 -> Mux4/10
  [P_D] -> Sum22/1
  Demux5/12 -> Mux4/12
  Demux5/8 -> Mux4/8
  Demux5/6 -> Sum24/2
  Demux5/7 -> Mux4/7
  Demux5/4 -> Sum22/2
  Sum24/1 -> Mux4/6
  [Y_D] -> Sum24/1
  Demux5/1 -> Mux4/1
  Sum22/1 -> Mux4/4
  Demux5/3 -> Mux4/3
  Demux5/2 -> Mux4/2
  Demux5/5 -> Sum23/2
  Mux4/1 -> Gain6/1, Gain5/1, Gain4/1
  [R_D] -> Sum26/1
  Sum26/1 -> Mux5/5
  Demux6/11 -> Mux5/11
  Demux6/9 -> Mux5/9
  Demux6/10 -> Mux5/10
  [P_D] -> Sum25/1
  Demux6/12 -> Mux5/12
  Demux6/8 -> Mux5/8
  Demux6/6 -> Sum27/2
  Demux6/7 -> Mux5/7
  Demux6/4 -> Sum25/2
  Sum27/1 -> Mux5/6
  [Y_D] -> Sum27/1
  Demux6/1 -> Mux5/1
  Sum25/1 -> Mux5/4
  Demux6/3 -> Mux5/3
  Demux6/2 -> Mux5/2
  Demux6/5 -> Sum26/2
  Mux5/1 -> Gain9/1, Gain8/1
  Step1/1 -> Switch1/2
  Step3/1 -> Switch2/2
  Transport Delay3/1 -> Switch1/1
  Step2/1 -> Switch3/1
  Ramp1/1 -> Sum28/2
  Constant1/1 -> Switch1/3, Switch2/3, Switch3/3
  Step/1 -> Switch3/2, Switch/2
  Ramp/1 -> Sum28/1
  Transport Delay4/1 -> Switch2/1
  Sine Wave1/1 -> Transport Delay3/1
  Step6/1 -> Switch/1
  Sum28/1 -> Switch/3
  Sine Wave3/1 -> Transport Delay4/1
  Step5/1 -> Goto25/1
  Constant6/1 -> Goto24/1, Goto21/1, Goto23/1
  Switch/1 -> Scope13/1, [Z_CMD]  "Z_CMD"
  Switch1/1 -> Scope13/2, [PT_CMD]  "PT_CMD"
  Switch2/1 -> Scope13/3, [RT_CMD]  "RT_CMD"
  Switch3/1 -> Scope13/4, [Yaw_CMD]  "YT_CMD"
  Transport Delay/1 -> [P_D]
  Transport Delay1/1 -> [R_D]
  Transport Delay2/1 -> [Y_D]
  [Yaw_LQR] -> Scope11/3
  [Roll_LQR] -> Scope11/1
  [Roll_PID_ITAE] -> Scope10/1
  [Y_LQR_OBS] -> Scope9/2  "Y, LQR-OBS"
  [X_LQR_OBS] -> Scope9/1  "X, LQR-OBS"
  [Pitch_LQR] -> Scope11/2
  [Roll_LQR_OBS] -> Scope12/1
  [Z_LQR_OBS] -> Scope9/3
  [Z_PID_ITAE] -> Scope5/3
  [Pitch_LQR_OBS] -> Scope12/2
  [X_LQR] -> Scope6/1  "X, LQR"
  [Y_LQR] -> Scope6/2  "Y, LQR"
  [Z_LQR] -> Scope6/3
  [Pitch_PID_ITAE] -> Scope10/2
  [Y_PID_ITAE] -> Scope5/2  "Y, PID-ITAE"
  [Yaw_LQR_OBS] -> Scope12/3
  [Yaw_PID_ITAE] -> Scope10/3
  [X_PID_ITAE] -> Scope5/1  "X, PID-ITAE"
